simulink library "pi_ctrl"  (R2017b)
settings: Solver=VariableStepAuto  StartTime=0.0  StopTime=10.0  RelTol=1e-3
undefined symbols (not defined in the file or in its folder): DiscIntNeverNeededParam, Int_init, Tctrl
settings Model: Creator=pkoralew  LastModifiedBy=pkoralew

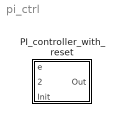
== system pi_ctrl ==
  PI_controller_with_reset : Subsystem  mask{Kp=0.4, Ti=40e-3, Ts=Tctrl, Iup=1.5, Idown=0, PIup=1.5, PIdown=0}
      mask prompts: Kp "Proportional gain Kp"; Ti "Integral doubling-time Ti [s]"; Ts "Sample time [s]"; Iup "Integral upper saturation limit"; Idown "Integral lower saturation limit"; PIup "PI output upper saturation limit"; PIdown "PI output lower saturation limit"
      mask help: PID controller integral is in enable state when Enable signal value equals 1. If Enable state equals zero the PID output also equals zero.

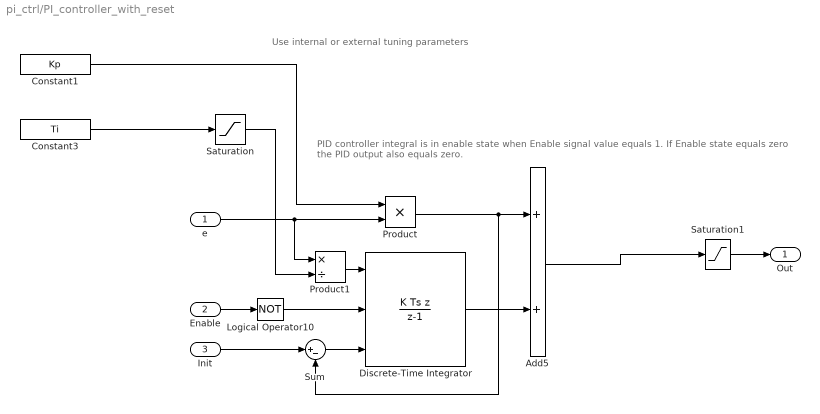
== system pi_ctrl/PI_controller_with_reset ==
  note: Use internal or external tuning parameters
  note: PID controller integral is in enable state when Enable signal value equals 1. If Enable state equals zero the PID output also equals zero.
  e : Inport
  Enable : Inport  Port=2
  Init : Inport  Port=3
  Add5 : Sum
  Constant1 : Constant  Value=Kp
  Constant3 : Constant  Value=Ti
  Discrete-Time Integrator : DiscreteIntegrator  IntegratorMethod=Integration: Backward Euler  gainval=1  ExternalReset=level  InitialConditionSource=external  InitialCondition=Int_init  SampleTime=Ts  LimitOutput=on  UpperSaturationLimit=Iup  LowerSaturationLimit=Idown  ICPrevOutput=DiscIntNeverNeededParam  ICPrevScaledInput=DiscIntNeverNeededParam
  Logical Operator10 : Logic  Operator=NOT  IconShape=distinctive  AllPortsSameDT=off  OutDataTypeStr=boolean
  Product : Product
  Product1 : Product  Inputs=*/
  Saturation : Saturate  UpperLimit=inf  LowerLimit=0.0001
  Saturation1 : Saturate  UpperLimit=PIup  LowerLimit=PIdown  LinearizeAsGain=off
  Sum : Sum  Inputs=|+-
  Out : Outport
  wires:
  Saturation1/1 -> Out/1
  Add5/1 -> Saturation1/1
  Enable/1 -> Logical Operator10/1
  Product/1 -> Sum/2, Add5/1
  Discrete-Time Integrator/1 -> Add5/2
  e/1 -> Product/2, Product1/1
  Logical Operator10/1 -> Discrete-Time Integrator/2
  Constant1/1 -> Product/1
  Constant3/1 -> Saturation/1
  Product1/1 -> Discrete-Time Integrator/1
  Saturation/1 -> Product1/2
  Init/1 -> Sum/1
  Sum/1 -> Discrete-Time Integrator/3
